simulink model "Model2"  (R2024b)
settings: Solver=ode4  StartTime=0.0  StopTime=100  FixedStep=0.01  RelTol=1e-3
values from neighbouring files (symbols this model uses):
  ARM_P_PID = [10 0 20]*0.1    [Single_ARM_Monte.m]    (also in main_starter.m)
  ARM_T_PID = [100 0 0]    [Single_ARM_Monte.m]    (also in main_starter.m)
  ARM_V_PID = [10 0 5]*0.1    [Single_ARM_Monte.m]    (also in main_starter.m)
  D_Joint0_angle0 = 45    [Single_ARM_Monte.m]    (also in main_starter.m)
  D_Joint0_angle1 = 0    [Single_ARM_Monte.m]    (also in main_starter.m)
  D_Joint0_angle2 = 0    [Single_ARM_Monte.m]    (also in main_starter.m)
  D_Joint0_rate0 = 0    [Single_ARM_Monte.m]    (also in main_starter.m)
  D_Joint0_rate1 = 0    [Single_ARM_Monte.m]    (also in main_starter.m)
  D_Joint0_rate2 = 0    [Single_ARM_Monte.m]    (also in main_starter.m)
  Joint_Motor_Mass = 23    [Single_ARM_Monte.m]    (also in main_starter.m)
  L_Joint0_angle0 = 45    [Single_ARM_Monte.m]    (also in main_starter.m)
  L_Joint0_angle1 = 0    [Single_ARM_Monte.m]    (also in main_starter.m)
  L_Joint0_angle2 = 0    [Single_ARM_Monte.m]    (also in main_starter.m)
  L_Joint0_rate0 = 0    [Single_ARM_Monte.m]    (also in main_starter.m)
  L_Joint0_rate1 = 0    [Single_ARM_Monte.m]    (also in main_starter.m)
  L_Joint0_rate2 = 0    [Single_ARM_Monte.m]    (also in main_starter.m)
  L_Joint_Offset = [ ... (first row only)    [Single_ARM_Monte.m]    (also in main_starter.m)
  Link1_Mass = 11    [Single_ARM_Monte.m]    (also in main_starter.m)
  Link2_Mass = 15.6    [Single_ARM_Monte.m]    (also in main_starter.m)
  Link3_Mass = 11    [Single_ARM_Monte.m]    (also in main_starter.m)
  Motor_transfer_Den = [1 100]    [Single_ARM_Monte.m]    (also in main_starter.m)
  Motor_transfer_Num = [100]    [Single_ARM_Monte.m]    (also in main_starter.m)
  PID_dt = 0.01    [Single_ARM_Monte.m]    (also in main_starter.m)
  R_Joint0_angle0 = 45    [Single_ARM_Monte.m]    (also in main_starter.m)
  R_Joint0_angle1 = 0    [Single_ARM_Monte.m]    (also in main_starter.m)
  R_Joint0_angle2 = 0    [Single_ARM_Monte.m]    (also in main_starter.m)
  R_Joint0_rate0 = 0    [Single_ARM_Monte.m]    (also in main_starter.m)
  R_Joint0_rate1 = 0    [Single_ARM_Monte.m]    (also in main_starter.m)
  R_Joint0_rate2 = 0    [Single_ARM_Monte.m]    (also in main_starter.m)
  RW_Att_D = 0.5    [Single_ARM_Monte.m]    (also in main_starter.m)
  RW_Att_I = 0.2    [Single_ARM_Monte.m]    (also in main_starter.m)
  RW_Att_P = 0.1    [Single_ARM_Monte.m]    (also in main_starter.m)
  RW_Mass = 100    [Single_ARM_Monte.m]    (also in main_starter.m)
  S_Body_Mass = 5    [Single_ARM_Monte.m]    (also in main_starter.m)
  S_init_pos = [0 0 0]'    [Single_ARM_Monte.m]    (also in main_starter.m)
  S_init_vel = [0 0 0]'    [Single_ARM_Monte.m]    (also in main_starter.m)
  T_Body_Mass = 4    [Single_ARM_Monte.m]    (also in main_starter.m)
  T_init_pos = [T_init_pos_list(i,1) T_init_pos_list(i,2) 0]'    [Single_ARM_Monte.m]    (also in main_starter.m = [1 0 0]')
  T_init_vel = [0 0 0]'    [Single_ARM_Monte.m]    (also in main_starter.m)
  Torq_mea_transfer_Den = [1 5]    [Single_ARM_Monte.m]    (also in main_starter.m)
  Torq_mea_transfer_Num = [5]    [Single_ARM_Monte.m]    (also in main_starter.m)
  U_Joint0_angle0 = 45    [Single_ARM_Monte.m]    (also in main_starter.m)
  U_Joint0_angle1 = 0    [Single_ARM_Monte.m]    (also in main_starter.m)
  U_Joint0_angle2 = 0    [Single_ARM_Monte.m]    (also in main_starter.m)
  U_Joint0_rate0 = 0    [Single_ARM_Monte.m]    (also in main_starter.m)
  U_Joint0_rate1 = 0    [Single_ARM_Monte.m]    (also in main_starter.m)
  U_Joint0_rate2 = 0    [Single_ARM_Monte.m]    (also in main_starter.m)
undefined symbols (not defined in the file or in its folder): X, Y, Z
libraries: nesl_utility x315, sm_lib x282, simulink_extras x46, sharedtransform x25, aerolibutil x4, simulink x2, matrix_library x2, dspmtrx3 x1
(part 12 of 12)

== matlab function Model2/Quad_ARM_Simplify/Down_ARM/MATLAB Function6 ==
  settings: updateMethod=DISCRETE
  data: cmd input; t_cmd output; cmd_d input; t_mea input; vd_mea input; v_mea input; p_mea input; mode input; tc_gain input; vc_gain input; pc_gain input; dt input
function t_cmd = motor_control(cmd,cmd_d, t_mea, vd_mea, v_mea, p_mea, mode, tc_gain, vc_gain, pc_gain, dt)

persistent I_save
persistent first_flg

if isempty(first_flg)
    I_save = 0;
    first_flg = 1;
end

if(mode == 1)%torque control
    % cmd : torque command [Nm]
    kp = tc_gain(1);
    ki = tc_gain(2);
    err = cmd - t_mea;
    t_cmd = kp*(cmd - t_mea) + ki*I_save;
    I_save = I_save + err*dt;

elseif(mode == 2) %velocity control
    % cmd : velocity command [rad/s]
    kp = vc_gain(1);
    % ki = vc_gain(2);
    kd = vc_gain(3);

    err = cmd - v_mea;
    errd = cmd_d - vd_mea;
    % t_cmd = (kp*err) + (kd*errd);
    t_cmd = (kp*err) + (kd*errd);
elseif(mode == 3) %position control : position command [rad]
    kp = pc_gain(1);
    % ki = pc_gain(2);
    kd = pc_gain(3);

    err = cmd - p_mea;
    errd = cmd_d - v_mea;
    t_cmd = (kp*err) + (kd*errd);
else%torque control
    t_cmd = 0;
end



end

== matlab function Model2/Quad_ARM_Simplify/Down_ARM/MATLAB Function7 ==
  data: v_sig input; v_out output; vd_out output; vd_sig input; t_mea input
function [v_out, vd_out] = limit_checker(v_sig,vd_sig,  t_mea)


if(abs(t_mea)>=0.01)
    vd_out = 0;
    v_out = 0;
else
    vd_out = vd_sig;
    v_out = v_sig;
end




end

== matlab function Model2/Quad_ARM_Simplify/End_Position_Flg ==
  data: L_J input; res output; R_J input; U_J input; D_J input
function res  = Motion_CMD(L_J, R_J, U_J, D_J)

deg2rad = 0.017453292519943;
rad2deg = 57.295779513082323;

L_END_FLG = 0;
R_END_FLG = 0;
U_END_FLG = 0;
D_END_FLG = 0;

Limit_Angle0 =     9.425*deg2rad;
Limit_Angle1 =   71.133*deg2rad;
Limit_Angle2 = 106.792*deg2rad;


L_END_FLG = End_Checker(L_J, [Limit_Angle0,-Limit_Angle1,-Limit_Angle2]);
R_END_FLG = End_Checker(R_J, [-Limit_Angle0,Limit_Angle1,Limit_Angle2]);
U_END_FLG = End_Checker(U_J, [-Limit_Angle0,Limit_Angle1,Limit_Angle2]);
D_END_FLG = End_Checker(D_J, [Limit_Angle0,-Limit_Angle1,-Limit_Angle2]);

res = [L_END_FLG,R_END_FLG,U_END_FLG,D_END_FLG]';

end

function res = End_Checker (Joint_Angle, Limit_Angle)

Limit_J0 = Limit_Angle(1);
Limit_J1 = Limit_Angle(2);
Limit_J2 = Limit_Angle(3);

J0 = Joint_Angle(1);
J1 = Joint_Angle(2);
J2 = Joint_Angle(3);

del = 5*pi/180;

J0_flg = 0; J1_flg = 0; J2_flg = 0;

if ((J0 <= (Limit_J0+del)) && (J0 >= (Limit_J0-del)))
    J0_flg = 1;
else
    J0_flg = 0;
end

if ((J1 <= (Limit_J1+del)) && (J1 >= (Limit_J1-del)))
    J1_flg = 1;
else
    J1_flg = 0;
end

if ((J2 <= (Limit_J2+del)) && (J2 >= (Limit_J2-del)))
    J2_flg = 1;
else
    J2_flg = 0;
end

if (J0_flg && J1_flg && J2_flg)
    res = 1;
else
    res = 0;
end

end

== matlab function Model2/Quad_ARM_Simplify/Fabrik_based_EE_Control(Angle) ==
  data: target input; q_list output; tol input; pos_list output; max_iter input; iter_fin output
function [q_list, pos_list, iter_fin] = fabrik_3link(target, tol, max_iter)
% target: [x; y] 목표 위치
% L: [L1, L2, L3] 링크 길이
% tol: 허용 오차 (예: 1e-4)
% max_iter: 반복 한계 (예: 100)

L = ...
[sqrt(0.04494^2 + 0.08979^2);
 0.1665;
 sqrt(0.02945^2 + 0.1232^2)];


[positions, ee_pose] = fk_3link([50,0,0]'*pi/180, L(1), L(2), L(3));

% 초기 관절 위치 (x, y) 초기화
pos_list = zeros(2, 4); % P0, P1, P2, P3
pos_list(:,1) = [0; 0];                    % Base
pos_list(:,2) = positions(:,1) + [L(1); 0]; % P1
pos_list(:,3) = positions(:,2) + [L(2); 0]; % P2
pos_list(:,4) = positions(:,3) + [L(3); 0]; % EE (초기화)

% Base 저장
base = pos_list(:,1);

% 목표 거리
total_length = sum(L);
if norm(target - base) > total_length
    % error("목표가 작업공간을 벗어났습니다.");
    target = total_length*(target/norm(target));
end

iter_fin = 0;

for iter = 1:max_iter
    % 1. FORWARD REACHING
    pos_list(:,4) = target; % 끝단 고정
    for i = 3:-1:1
        r = norm(pos_list(:,i+1) - pos_list(:,i));
        lambda = L(i) / r;
        pos_list(:,i) = (1 - lambda) * pos_list(:,i+1) + lambda * pos_list(:,i);
    end

    % 2. BACKWARD REACHING
    pos_list(:,1) = base; % base 고정
    for i = 1:3
        r = norm(pos_list(:,i+1) - pos_list(:,i));
        lambda = L(i) / r;
        pos_list(:,i+1) = (1 - lambda) * pos_list(:,i) + lambda * pos_list(:,i+1);
    end

    % 3. 수렴 확인
    err = norm(pos_list(:,end) - target);
    if err < tol
        break;
    end
    iter_fin = iter;
end

% P0 = joint_pos(:,1); P1 = joint_pos(:,2);
P2 = pos_list(:,2); P3 = pos_list(:,3);
% P4 = joint_pos(:,5); 
P5 = pos_list(:,4);

t0 = atan2(P2(2), P2(1));
temp = P3 - P2;
t1 = atan2(temp(2), temp(1)) - t0;
temp = P5 - P3;
t2 = atan2(temp(2), temp(1)) - t0 - t1;



q_list = [t0,t1,t2]';

end

function [positions, ee_pose] = fk_3link(theta, a1, a2, a3)
    % theta: [theta1, theta2, theta3] (rad)
    % a1, a2, a3: 링크 길이
    % positions: [P0; P1; P2; P3] (각 조인트 위치)
    % ee_pose: [x, y, phi] (EE 위치 + 자세)

    theta1 = theta(1);
    theta2 = theta(2);
    theta3 = theta(3);

    % 누적 각도
    t1 = theta1;
    t2 = theta1 + theta2;
    t3 = t2 + theta3;

    % 각 조인트 위치 계산
    P0 = [0; 0];
    P1 = P0 + a1 * [cos(t1); sin(t1)];
    P2 = P1 + a2 * [cos(t2); sin(t2)];
    P3 = P2 + a3 * [cos(t3); sin(t3)];

    % 자세
    phi = t3;

    % 출력
    positions = [P0, P1, P2, P3];  % 각 열이 각 위치
    ee_pose = [P3(1), P3(2)]'; % EE 위치 및 방향
end

== matlab function Model2/Single_ARM/MATLAB Function ==
  data: theta input; pos output
function pos = fk_3link_explicit(theta)
    L0 = 0.04494;
    L1 = 0.08979;
    L2 = 0.1665;
    L3a = 0.02945;
    L3b = 0.1232;

    t0 = theta(1);
    t1 = theta(2);
    t2 = theta(3);
    t01 = t0 + t1;
    t012 = t01 + t2;

    R = @(theta) [cos(theta); sin(theta)];

    P0 = [0; 0];
    P1 = P0 + L0 * R(t0 + pi/2);
    P2 = P1 + L1 * R(t0);
    P3 = P2 + L2 * R(t01);
    P4 = P3 + L3a * R(t012 + pi/2);
    pos = P4 + L3b * R(t012);  % EE 위치
end

== matlab function Model2/Quad_ARM_Simplify/Jacobian_based_EE_Control(Rate) ==
  data: q input; qd_cmd output; target_pos input
function qd_cmd = Jacobian_based_EE_Control(q, target_pos)
% target_pos = [0.3 0 0]';
pos = fk_3link_explicit(q);
J = jacobian_3link(q);

L = ...
[sqrt(0.04494^2 + 0.08979^2);
 0.1665;
 sqrt(0.02945^2 + 0.1232^2)];

% 목표 거리
total_length = sum(L);
if norm(target_pos) > total_length
    % error("목표가 작업공간을 벗어났습니다.");
    target_pos = total_length*(target_pos/norm(target_pos));
end

err = 2*(target_pos - pos);
Z = 0*[1 1 1]';
qd_cmd = pinv(J)*err + (eye(3,3) - pinv(J)*J)*Z;

end

function pos = fk_3link_explicit(theta)
    L0 = 0.04494;
    L1 = 0.08979;
    L2 = 0.1665;
    L3a = 0.02945;
    L3b = 0.1232;

    t0 = theta(1);
    t1 = theta(2);
    t2 = theta(3);
    t01 = t0 + t1;
    t012 = t01 + t2;

    R = @(theta) [cos(theta); sin(theta)];

    P0 = [0; 0];
    P1 = P0 + L0 * R(t0 + pi/2);
    P2 = P1 + L1 * R(t0);
    P3 = P2 + L2 * R(t01);
    P4 = P3 + L3a * R(t012 + pi/2);
    pos = P4 + L3b * R(t012);  % EE 위치
end

function J = jacobian_3link(theta)
    L0 = 0.04494;
    L1 = 0.08979;
    L2 = 0.1665;
    L3a = 0.02945;
    L3b = 0.1232;

    t0 = theta(1);
    t1 = theta(2);
    t2 = theta(3);
    t01 = t0 + t1;
    t012 = t01 + t2;

    Rp = @(theta) [-sin(theta); cos(theta)]; 

    J1 =  L0 * Rp(t0 + pi/2) ...
         +L1 * Rp(t0) ...
         +L2 * Rp(t01) ...
         +L3a * Rp(t012 + pi/2) ...
         +L3b * Rp(t012);

    J2 =  L2 * Rp(t01) ...
         +L3a * Rp(t012 + pi/2) ...
         +L3b * Rp(t012);

    J3 =  L3a * Rp(t012 + pi/2) ...
         +L3b * Rp(t012);

    J = [J1, J2, J3];
end

== matlab function Model2/Quad_ARM_Simplify/Left_ARM/MATLAB Function2 ==
  settings: updateMethod=DISCRETE
  data: cmd input; t_cmd output; cmd_d input; t_mea input; vd_mea input; v_mea input; p_mea input; mode input; tc_gain input; vc_gain input; pc_gain input; dt input
function t_cmd = motor_control(cmd, cmd_d, t_mea, vd_mea, v_mea, p_mea, mode, tc_gain, vc_gain, pc_gain, dt)

persistent I_save
persistent first_flg

if isempty(first_flg)
    I_save = 0;
    first_flg = 1;
end

if(mode == 1)%torque control
    % cmd : torque command [Nm]
    kp = tc_gain(1);
    ki = tc_gain(2);
    err = cmd - t_mea;
    t_cmd = kp*(cmd - t_mea) + ki*I_save;
    I_save = I_save + err*dt;

elseif(mode == 2) %velocity control
    % cmd : velocity command [rad/s]
    kp = vc_gain(1);
    % ki = vc_gain(2);
    kd = vc_gain(3);

    err = cmd - v_mea;
    errd = cmd_d - vd_mea;
    % t_cmd = (kp*err) + (kd*errd);
    t_cmd = (kp*err) + (kd*errd);
elseif(mode == 3) %position control : position command [rad]
    kp = pc_gain(1);
    % ki = pc_gain(2);
    kd = pc_gain(3);

    err = cmd - p_mea;
    errd = cmd_d - v_mea;
    t_cmd = (kp*err) + (kd*errd);
else%torque control
    t_cmd = 0;
end



end

== matlab function Model2/Quad_ARM_Simplify/Left_ARM/MATLAB Function3 ==
  data: v_sig input; v_out output; vd_out output; vd_sig input; t_mea input
function [v_out, vd_out] = limit_checker(v_sig,vd_sig,  t_mea)


if(abs(t_mea)>=0.01)
    vd_out = 0;
    v_out = 0;
else
    vd_out = vd_sig;
    v_out = v_sig;
end




end

== matlab function Model2/Quad_ARM_Simplify/Left_ARM/MATLAB Function4 ==
  settings: updateMethod=DISCRETE
  data: cmd input; t_cmd output; cmd_d input; t_mea input; vd_mea input; v_mea input; p_mea input; mode input; tc_gain input; vc_gain input; pc_gain input; dt input
function t_cmd = motor_control(cmd,cmd_d, t_mea, vd_mea, v_mea, p_mea, mode, tc_gain, vc_gain, pc_gain, dt)

persistent I_save
persistent first_flg

if isempty(first_flg)
    I_save = 0;
    first_flg = 1;
end

if(mode == 1)%torque control
    % cmd : torque command [Nm]
    kp = tc_gain(1);
    ki = tc_gain(2);
    err = cmd - t_mea;
    t_cmd = kp*(cmd - t_mea) + ki*I_save;
    I_save = I_save + err*dt;

elseif(mode == 2) %velocity control
    % cmd : velocity command [rad/s]
    kp = vc_gain(1);
    % ki = vc_gain(2);
    kd = vc_gain(3);

    err = cmd - v_mea;
    errd = cmd_d - vd_mea;
    % t_cmd = (kp*err) + (kd*errd);
    t_cmd = (kp*err) + (kd*errd);
elseif(mode == 3) %position control : position command [rad]
    kp = pc_gain(1);
    ki = pc_gain(2);
    kd = pc_gain(3);

    err = cmd - p_mea;
    errd = cmd_d - v_mea;
    t_cmd = (kp*err) + (kd*errd);
else%torque control
    t_cmd = 0;
end



end

== matlab function Model2/Quad_ARM_Simplify/Left_ARM/MATLAB Function5 ==
  data: v_sig input; v_out output; vd_out output; vd_sig input; t_mea input
function [v_out, vd_out] = limit_checker(v_sig,vd_sig,  t_mea)


if(abs(t_mea)>=0.01)
    vd_out = 0;
    v_out = 0;
else
    vd_out = vd_sig;
    v_out = v_sig;
end




end

== matlab function Model2/Quad_ARM_Simplify/Left_ARM/MATLAB Function6 ==
  settings: updateMethod=DISCRETE
  data: cmd input; t_cmd output; cmd_d input; t_mea input; vd_mea input; v_mea input; p_mea input; mode input; tc_gain input; vc_gain input; pc_gain input; dt input
function t_cmd = motor_control(cmd,cmd_d, t_mea, vd_mea, v_mea, p_mea, mode, tc_gain, vc_gain, pc_gain, dt)

persistent I_save
persistent first_flg

if isempty(first_flg)
    I_save = 0;
    first_flg = 1;
end

if(mode == 1)%torque control
    % cmd : torque command [Nm]
    kp = tc_gain(1);
    ki = tc_gain(2);
    err = cmd - t_mea;
    t_cmd = kp*(cmd - t_mea) + ki*I_save;
    I_save = I_save + err*dt;

elseif(mode == 2) %velocity control
    % cmd : velocity command [rad/s]
    kp = vc_gain(1);
    % ki = vc_gain(2);
    kd = vc_gain(3);

    err = cmd - v_mea;
    errd = cmd_d - vd_mea;
    % t_cmd = (kp*err) + (kd*errd);
    t_cmd = (kp*err) + (kd*errd);
elseif(mode == 3) %position control : position command [rad]
    kp = pc_gain(1);
    % ki = pc_gain(2);
    kd = pc_gain(3);

    err = cmd - p_mea;
    errd = cmd_d - v_mea;
    t_cmd = (kp*err) + (kd*errd);
else%torque control
    t_cmd = 0;
end



end

== matlab function Model2/Single_ARM/MATLAB Function2 ==
  settings: updateMethod=DISCRETE
  data: cmd input; t_cmd output; cmd_d input; t_mea input; vd_mea input; v_mea input; p_mea input; mode input; tc_gain input; vc_gain input; pc_gain input; dt input
function t_cmd = motor_control(cmd,cmd_d, t_mea, vd_mea, v_mea, p_mea, mode, tc_gain, vc_gain, pc_gain, dt)

persistent I_save
persistent first_flg

if isempty(first_flg)
    I_save = 0;
    first_flg = 1;
end

if(mode == 1)%torque control
    % cmd : torque command [Nm]
    kp = tc_gain(1);
    ki = tc_gain(2);
    err = cmd - t_mea;
    t_cmd = kp*(cmd - t_mea) + ki*I_save;
    I_save = I_save + err*dt;

elseif(mode == 2) %velocity control
    % cmd : velocity command [rad/s]
    kp = vc_gain(1);
    % ki = vc_gain(2);
    kd = vc_gain(3);

    err = cmd - v_mea;
    errd = cmd_d - vd_mea;
    % t_cmd = (kp*err) + (kd*errd);
    t_cmd = (kp*err) + (kd*errd);
elseif(mode == 3) %position control : position command [rad]
    kp = pc_gain(1);
    % ki = pc_gain(2);
    kd = pc_gain(3);

    err = cmd - p_mea;
    errd = cmd_d - v_mea;
    t_cmd = (kp*err) + (kd*errd);
else%torque control
    t_cmd = 0;
end



end

== matlab function Model2/Quad_ARM_Simplify/Left_ARM/MATLAB Function7 ==
  data: v_sig input; v_out output; vd_out output; vd_sig input; t_mea input
function [v_out, vd_out] = limit_checker(v_sig,vd_sig,  t_mea)


if(abs(t_mea)>=0.01)
    vd_out = 0;
    v_out = 0;
else
    vd_out = vd_sig;
    v_out = v_sig;
end




end

== matlab function Model2/Quad_ARM_Simplify/MATLAB Function ==
  data: theta input; pos output
function pos = fk_3link_explicit(theta)
    L0 = 0.04494;
    L1 = 0.08979;
    L2 = 0.1665;
    L3a = 0.02945;
    L3b = 0.1232;

    t0 = theta(1);
    t1 = theta(2);
    t2 = theta(3);
    t01 = t0 + t1;
    t012 = t01 + t2;

    R = @(theta) [cos(theta); sin(theta)];

    P0 = [0; 0];
    P1 = P0 + L0 * R(t0 + pi/2);
    P2 = P1 + L1 * R(t0);
    P3 = P2 + L2 * R(t01);
    P4 = P3 + L3a * R(t012 + pi/2);
    pos = P4 + L3b * R(t012);  % EE 위치
end

== matlab function Model2/Quad_ARM_Simplify/MATLAB Function1 ==
  data: theta input; J output
function J = jacobian_3link(theta)
    L0 = 0.04494;
    L1 = 0.08979;
    L2 = 0.1665;
    L3a = 0.02945;
    L3b = 0.1232;

    t0 = theta(1);
    t1 = theta(2);
    t2 = theta(3);
    t01 = t0 + t1;
    t012 = t01 + t2;

    Rp = @(theta) [-sin(theta); cos(theta)]; 

    J1 =  L0 * Rp(t0 + pi/2) ...
         +L1 * Rp(t0) ...
         +L2 * Rp(t01) ...
         +L3a * Rp(t012 + pi/2) ...
         +L3b * Rp(t012);

    J2 =  L2 * Rp(t01) ...
         +L3a * Rp(t012 + pi/2) ...
         +L3b * Rp(t012);

    J3 =  L3a * Rp(t012 + pi/2) ...
         +L3b * Rp(t012);

    J = [J1, J2, J3];
end

== matlab function Model2/Quad_ARM_Simplify/MATLAB Function2 ==
  data: u input; y output
function y = fcn(u)

y = u(:,4);

end

== matlab function Model2/Quad_ARM_Simplify/MATLAB Function3 ==
  data: theta input; pos output
function pos = fk_3link_explicit(theta)
    L0 = 0.04494;
    L1 = 0.08979;
    L2 = 0.1665;
    L3a = 0.02945;
    L3b = 0.1232;

    t0 = theta(1);
    t1 = theta(2);
    t2 = theta(3);
    t01 = t0 + t1;
    t012 = t01 + t2;

    R = @(theta) [cos(theta); sin(theta)];

    P0 = [0; 0];
    P1 = P0 + L0 * R(t0 + pi/2);
    P2 = P1 + L1 * R(t0);
    P3 = P2 + L2 * R(t01);
    P4 = P3 + L3a * R(t012 + pi/2);
    pos = P4 + L3b * R(t012);  % EE 위치
end

== matlab function Model2/Quad_ARM_Simplify/MATLAB Function5 ==
  data: theta input; pos output
function pos = fk_3link_explicit(theta)
    L0 = 0.04494;
    L1 = 0.08979;
    L2 = 0.1665;
    L3a = 0.02945;
    L3b = 0.1232;

    t0 = theta(1);
    t1 = theta(2);
    t2 = theta(3);
    t01 = t0 + t1;
    t012 = t01 + t2;

    R = @(theta) [cos(theta); sin(theta)];

    P0 = [0; 0];
    P1 = P0 + L0 * R(t0 + pi/2);
    P2 = P1 + L1 * R(t0);
    P3 = P2 + L2 * R(t01);
    P4 = P3 + L3a * R(t012 + pi/2);
    pos = P4 + L3b * R(t012);  % EE 위치
end

== matlab function Model2/Quad_ARM_Simplify/MATLAB Function6 ==
  data: theta input; positions output; ee_pose output
function [positions, ee_pose] = fk_3link_simplify(theta)
    % theta: [theta1, theta2, theta3] (rad)
    % a1, a2, a3: 링크 길이
    % positions: [P0; P1; P2; P3] (각 조인트 위치)
    % ee_pose: [x, y, phi] (EE 위치 + 자세)

    L = [sqrt(0.04494^2 + 0.08979^2);
           0.1665;
           sqrt(0.02945^2 + 0.1232^2)];

    theta1 = theta(1);
    theta2 = theta(2);
    theta3 = theta(3);

    % 누적 각도
    t1 = theta1;
    t2 = theta1 + theta2;
    t3 = t2 + theta3;

    % 각 조인트 위치 계산
    P0 = [0; 0];
    P1 = P0 + L(1) * [cos(t1); sin(t1)];
    P2 = P1 + L(2) * [cos(t2); sin(t2)];
    P3 = P2 + L(3) * [cos(t3); sin(t3)];

    % 자세
    phi = t3;

    % 출력
    positions = [P0, P1, P2, P3];  % 각 열이 각 위치
    ee_pose = [P3(1), P3(2)]'; % EE 위치 및 방향
end

== matlab function Model2/Quad_ARM_Simplify/Openning_Motion_Sequence ==
  data: b_flg input; res output; mode output
function [res, mode] = Motion_CMD(b_flg)

deg2rad = pi/180;

% if (t <= 10)
%     res = [45 -90 -180]'*deg2rad;
% 
% elseif ((t>=10) && (t<=20))
%     res = [45 0 -180]'*deg2rad;
% else
%     res = [45 0 0]'*deg2rad;
% end
% 
% mode = [3 3 3]';

Body_Contact_Total = (b_flg(1) == 1) && (b_flg(2) == 1) && (b_flg(3) == 1) && (b_flg(4) == 1);

if Body_Contact_Total
    res = [0 0 0]'*deg2rad;
    mode = [2 2 2]';
else
    res = [-4 -3 -4]'*deg2rad;
    mode = [2 2 2]';
end

end

== matlab function Model2/Quad_ARM_Simplify/Openning_Motion_Sequence1 ==
  data: t input; res output; mode output
function [res, mode] = Motion_CMD(t)

deg2rad = pi/180;

if (t <= 10)
    res = [45 -90 -180]'*deg2rad;

elseif ((t>=10) && (t<=20))
    res = [45 0 -180]'*deg2rad;
else
    res = [45 0 0]'*deg2rad;
end

mode = [3 3 3]';

end

== matlab function Model2/Quad_ARM_Simplify/Openning_Motion_Sequence2 ==
  data: b_flg input; res output; mode output
function [res, mode] = Motion_CMD(b_flg)

deg2rad = pi/180;

% if (t <= 10)
%     res = [45 -90 -180]'*deg2rad;
% 
% elseif ((t>=10) && (t<=20))
%     res = [45 0 -180]'*deg2rad;
% else
%     res = [45 0 0]'*deg2rad;
% end
% 
% mode = [3 3 3]';
% res = [-4 -3 -4]'*deg2rad;
% mode = [2 2 2]';
% res = [45 0 0]'*deg2rad;
% mode = [3 3 3]';
% 

Body_Contact_Total = (b_flg(1) == 1) && (b_flg(2) == 1) && (b_flg(3) == 1) && (b_flg(4) == 1);

if Body_Contact_Total
    res = [0 0 0]'*deg2rad;
    mode = [2 2 2]';
else
    res = [-4 -3 -4]'*deg2rad;
    mode = [2 2 2]';
end


end

== matlab function Model2/Quad_ARM_Simplify/Openning_Motion_Sequence3 ==
  data: b_flg input; res output; mode output
function [res, mode] = Motion_CMD(b_flg)

deg2rad = pi/180;

% res = [45 0 0]'*deg2rad;
% mode = [3 3 3]';


Body_Contact_Total = (b_flg(1) == 1) && (b_flg(2) == 1) && (b_flg(3) == 1) && (b_flg(4) == 1);

if Body_Contact_Total
    res = [0 0 0]'*deg2rad;
    mode = [2 2 2]';
else
    res = [-4 -3 -4]'*deg2rad;
    mode = [2 2 2]';
end

end

== matlab function Model2/Quad_ARM_Simplify/Openning_Motion_Sequence4 ==
  data: b_flg input; res output; mode output; pos_end_flg input
function [res, mode] = Motion_CMD(b_flg, pos_end_flg)

deg2rad = pi/180;

% res = [0 0 0]'*deg2rad;
% mode = [3 3 3]';


Body_Contact_Total = (b_flg(1) == 1) && (b_flg(2) == 1) && (b_flg(3) == 1) && (b_flg(4) == 1);
Pos_End_Total = pos_end_flg(1) && pos_end_flg(2) && pos_end_flg(3) && pos_end_flg(4);


if (Body_Contact_Total || Pos_End_Total)
    res = [0 0 0]'*deg2rad;
    mode = [2 2 2]';
else
    res = [-1 -2 -3]'*deg2rad;
    mode = [2 2 2]';
end

end

== matlab function Model2/Quad_ARM_Simplify/Right_ARM/MATLAB Function2 ==
  settings: updateMethod=DISCRETE
  data: cmd input; t_cmd output; cmd_d input; t_mea input; vd_mea input; v_mea input; p_mea input; mode input; tc_gain input; vc_gain input; pc_gain input; dt input
function t_cmd = motor_control(cmd, cmd_d, t_mea, vd_mea, v_mea, p_mea, mode, tc_gain, vc_gain, pc_gain, dt)

persistent I_save
persistent first_flg

if isempty(first_flg)
    I_save = 0;
    first_flg = 1;
end

if(mode == 1)%torque control
    % cmd : torque command [Nm]
    kp = tc_gain(1);
    ki = tc_gain(2);
    err = cmd - t_mea;
    t_cmd = kp*(cmd - t_mea) + ki*I_save;
    I_save = I_save + err*dt;

elseif(mode == 2) %velocity control
    % cmd : velocity command [rad/s]
    kp = vc_gain(1);
    % ki = vc_gain(2);
    kd = vc_gain(3);

    err = cmd - v_mea;
    errd = cmd_d - vd_mea;
    % t_cmd = (kp*err) + (kd*errd);
    t_cmd = (kp*err) + (kd*errd);
elseif(mode == 3) %position control : position command [rad]
    kp = pc_gain(1);
    % ki = pc_gain(2);
    kd = pc_gain(3);

    err = cmd - p_mea;
    errd = cmd_d - v_mea;
    t_cmd = (kp*err) + (kd*errd);
else%torque control
    t_cmd = 0;
end



end

== matlab function Model2/Quad_ARM_Simplify/Right_ARM/MATLAB Function3 ==
  data: v_sig input; v_out output; vd_out output; vd_sig input; t_mea input
function [v_out, vd_out] = limit_checker(v_sig,vd_sig,  t_mea)


if(abs(t_mea)>=0.01)
    vd_out = 0;
    v_out = 0;
else
    vd_out = vd_sig;
    v_out = v_sig;
end




end

== matlab function Model2/Quad_ARM_Simplify/Right_ARM/MATLAB Function4 ==
  settings: updateMethod=DISCRETE
  data: cmd input; t_cmd output; cmd_d input; t_mea input; vd_mea input; v_mea input; p_mea input; mode input; tc_gain input; vc_gain input; pc_gain input; dt input
function t_cmd = motor_control(cmd,cmd_d, t_mea, vd_mea, v_mea, p_mea, mode, tc_gain, vc_gain, pc_gain, dt)

persistent I_save
persistent first_flg

if isempty(first_flg)
    I_save = 0;
    first_flg = 1;
end

if(mode == 1)%torque control
    % cmd : torque command [Nm]
    kp = tc_gain(1);
    ki = tc_gain(2);
    err = cmd - t_mea;
    t_cmd = kp*(cmd - t_mea) + ki*I_save;
    I_save = I_save + err*dt;

elseif(mode == 2) %velocity control
    % cmd : velocity command [rad/s]
    kp = vc_gain(1);
    % ki = vc_gain(2);
    kd = vc_gain(3);

    err = cmd - v_mea;
    errd = cmd_d - vd_mea;
    % t_cmd = (kp*err) + (kd*errd);
    t_cmd = (kp*err) + (kd*errd);
elseif(mode == 3) %position control : position command [rad]
    kp = pc_gain(1);
    ki = pc_gain(2);
    kd = pc_gain(3);

    err = cmd - p_mea;
    errd = cmd_d - v_mea;
    t_cmd = (kp*err) + (kd*errd);
else%torque control
    t_cmd = 0;
end



end

== matlab function Model2/Quad_ARM_Simplify/Right_ARM/MATLAB Function5 ==
  data: v_sig input; v_out output; vd_out output; vd_sig input; t_mea input
function [v_out, vd_out] = limit_checker(v_sig,vd_sig,  t_mea)


if(abs(t_mea)>=0.01)
    vd_out = 0;
    v_out = 0;
else
    vd_out = vd_sig;
    v_out = v_sig;
end




end

== matlab function Model2/Quad_ARM_Simplify/Right_ARM/MATLAB Function6 ==
  settings: updateMethod=DISCRETE
  data: cmd input; t_cmd output; cmd_d input; t_mea input; vd_mea input; v_mea input; p_mea input; mode input; tc_gain input; vc_gain input; pc_gain input; dt input
function t_cmd = motor_control(cmd,cmd_d, t_mea, vd_mea, v_mea, p_mea, mode, tc_gain, vc_gain, pc_gain, dt)

persistent I_save
persistent first_flg

if isempty(first_flg)
    I_save = 0;
    first_flg = 1;
end

if(mode == 1)%torque control
    % cmd : torque command [Nm]
    kp = tc_gain(1);
    ki = tc_gain(2);
    err = cmd - t_mea;
    t_cmd = kp*(cmd - t_mea) + ki*I_save;
    I_save = I_save + err*dt;

elseif(mode == 2) %velocity control
    % cmd : velocity command [rad/s]
    kp = vc_gain(1);
    % ki = vc_gain(2);
    kd = vc_gain(3);

    err = cmd - v_mea;
    errd = cmd_d - vd_mea;
    % t_cmd = (kp*err) + (kd*errd);
    t_cmd = (kp*err) + (kd*errd);
elseif(mode == 3) %position control : position command [rad]
    kp = pc_gain(1);
    % ki = pc_gain(2);
    kd = pc_gain(3);

    err = cmd - p_mea;
    errd = cmd_d - v_mea;
    t_cmd = (kp*err) + (kd*errd);
else%torque control
    t_cmd = 0;
end



end

== matlab function Model2/Single_ARM/MATLAB Function3 ==
  data: v_sig input; v_out output; vd_out output; vd_sig input; t_mea input
function [v_out, vd_out] = limit_checker(v_sig,vd_sig,  t_mea)


if(abs(t_mea)>=0.5)
    vd_out = 0;
    v_out = 0;
else
    vd_out = vd_sig;
    v_out = v_sig;
end




end

== matlab function Model2/Quad_ARM_Simplify/Right_ARM/MATLAB Function7 ==
  data: v_sig input; v_out output; vd_out output; vd_sig input; t_mea input
function [v_out, vd_out] = limit_checker(v_sig,vd_sig,  t_mea)


if(abs(t_mea)>=0.01)
    vd_out = 0;
    v_out = 0;
else
    vd_out = vd_sig;
    v_out = v_sig;
end




end

== matlab function Model2/Quad_ARM_Simplify/Subsystem1/MATLAB Function1 ==
  data: qe input; Omegad output; we input; P_gain input; I_gain input; D_gain input; RW_config input
function Omegad = fcn(qe, we, P_gain, I_gain, D_gain, RW_config)

deg2rad = pi/180;

% beta = 63*deg2rad;

% RW1_axis = [cos(beta), 0, -sin(beta)]';
% RW3_axis = [-cos(beta), 0, -sin(beta)]';
% RW2_axis = [0, -cos(beta), sin(beta)]';
% RW4_axis = [0,  cos(beta), sin(beta)]';
% 
% RW_config = [RW1_axis, RW2_axis, RW3_axis, RW4_axis];

Kp = P_gain*diag([1 1 1]);
Kd = D_gain*diag([1 1 1]);

t = -(Kp*[qe(2); qe(3); qe(4)] + Kd*we);

Omegad = pinv(RW_config) * t;

end

function res = Rzyx(z,y,x)
   res = Rz(z)*Ry(y)*Rx(x);
end

function res = Rx(a)
% % % ang : rad
res = [1 0 0;
       0 cos(a) sin(a);
       0 -sin(a) cos(a)];
end

function res = Ry(a)
% % % ang : rad

res = [cos(a) 0 -sin(a);
                  0 1 0;
          sin(a) 0 cos(a)];

end

function res = Rz(a)
% % % ang : rad
res = [cos(a) sin(a) 0;
       -sin(a) cos(a) 0;
       0 0 1];

end

== matlab function Model2/Quad_ARM_Simplify/Up_ARM/MATLAB Function2 ==
  settings: updateMethod=DISCRETE
  data: cmd input; t_cmd output; cmd_d input; t_mea input; vd_mea input; v_mea input; p_mea input; mode input; tc_gain input; vc_gain input; pc_gain input; dt input
function t_cmd = motor_control(cmd, cmd_d, t_mea, vd_mea, v_mea, p_mea, mode, tc_gain, vc_gain, pc_gain, dt)

persistent I_save
persistent first_flg

if isempty(first_flg)
    I_save = 0;
    first_flg = 1;
end

if(mode == 1)%torque control
    % cmd : torque command [Nm]
    kp = tc_gain(1);
    ki = tc_gain(2);
    err = cmd - t_mea;
    t_cmd = kp*(cmd - t_mea) + ki*I_save;
    I_save = I_save + err*dt;

elseif(mode == 2) %velocity control
    % cmd : velocity command [rad/s]
    kp = vc_gain(1);
    % ki = vc_gain(2);
    kd = vc_gain(3);

    err = cmd - v_mea;
    errd = cmd_d - vd_mea;
    % t_cmd = (kp*err) + (kd*errd);
    t_cmd = (kp*err) + (kd*errd);
elseif(mode == 3) %position control : position command [rad]
    kp = pc_gain(1);
    % ki = pc_gain(2);
    kd = pc_gain(3);

    err = cmd - p_mea;
    errd = cmd_d - v_mea;
    t_cmd = (kp*err) + (kd*errd);
else%torque control
    t_cmd = 0;
end



end

== matlab function Model2/Quad_ARM_Simplify/Up_ARM/MATLAB Function3 ==
  data: v_sig input; v_out output; vd_out output; vd_sig input; t_mea input
function [v_out, vd_out] = limit_checker(v_sig,vd_sig,  t_mea)


if(abs(t_mea)>=0.01)
    vd_out = 0;
    v_out = 0;
else
    vd_out = vd_sig;
    v_out = v_sig;
end




end

== matlab function Model2/Quad_ARM_Simplify/Up_ARM/MATLAB Function4 ==
  settings: updateMethod=DISCRETE
  data: cmd input; t_cmd output; cmd_d input; t_mea input; vd_mea input; v_mea input; p_mea input; mode input; tc_gain input; vc_gain input; pc_gain input; dt input
function t_cmd = motor_control(cmd,cmd_d, t_mea, vd_mea, v_mea, p_mea, mode, tc_gain, vc_gain, pc_gain, dt)

persistent I_save
persistent first_flg

if isempty(first_flg)
    I_save = 0;
    first_flg = 1;
end

if(mode == 1)%torque control
    % cmd : torque command [Nm]
    kp = tc_gain(1);
    ki = tc_gain(2);
    err = cmd - t_mea;
    t_cmd = kp*(cmd - t_mea) + ki*I_save;
    I_save = I_save + err*dt;

elseif(mode == 2) %velocity control
    % cmd : velocity command [rad/s]
    kp = vc_gain(1);
    % ki = vc_gain(2);
    kd = vc_gain(3);

    err = cmd - v_mea;
    errd = cmd_d - vd_mea;
    % t_cmd = (kp*err) + (kd*errd);
    t_cmd = (kp*err) + (kd*errd);
elseif(mode == 3) %position control : position command [rad]
    kp = pc_gain(1);
    ki = pc_gain(2);
    kd = pc_gain(3);

    err = cmd - p_mea;
    errd = cmd_d - v_mea;
    t_cmd = (kp*err) + (kd*errd);
else%torque control
    t_cmd = 0;
end



end

== matlab function Model2/Quad_ARM_Simplify/Up_ARM/MATLAB Function5 ==
  data: v_sig input; v_out output; vd_out output; vd_sig input; t_mea input
function [v_out, vd_out] = limit_checker(v_sig,vd_sig,  t_mea)


if(abs(t_mea)>=0.01)
    vd_out = 0;
    v_out = 0;
else
    vd_out = vd_sig;
    v_out = v_sig;
end




end

== matlab function Model2/Quad_ARM_Simplify/Up_ARM/MATLAB Function6 ==
  settings: updateMethod=DISCRETE
  data: cmd input; t_cmd output; cmd_d input; t_mea input; vd_mea input; v_mea input; p_mea input; mode input; tc_gain input; vc_gain input; pc_gain input; dt input
function t_cmd = motor_control(cmd,cmd_d, t_mea, vd_mea, v_mea, p_mea, mode, tc_gain, vc_gain, pc_gain, dt)

persistent I_save
persistent first_flg

if isempty(first_flg)
    I_save = 0;
    first_flg = 1;
end

if(mode == 1)%torque control
    % cmd : torque command [Nm]
    kp = tc_gain(1);
    ki = tc_gain(2);
    err = cmd - t_mea;
    t_cmd = kp*(cmd - t_mea) + ki*I_save;
    I_save = I_save + err*dt;

elseif(mode == 2) %velocity control
    % cmd : velocity command [rad/s]
    kp = vc_gain(1);
    % ki = vc_gain(2);
    kd = vc_gain(3);

    err = cmd - v_mea;
    errd = cmd_d - vd_mea;
    % t_cmd = (kp*err) + (kd*errd);
    t_cmd = (kp*err) + (kd*errd);
elseif(mode == 3) %position control : position command [rad]
    kp = pc_gain(1);
    % ki = pc_gain(2);
    kd = pc_gain(3);

    err = cmd - p_mea;
    errd = cmd_d - v_mea;
    t_cmd = (kp*err) + (kd*errd);
else%torque control
    t_cmd = 0;
end



end

== matlab function Model2/Single_ARM/MATLAB Function4 ==
  settings: updateMethod=DISCRETE
  data: cmd input; t_cmd output; cmd_d input; t_mea input; vd_mea input; v_mea input; p_mea input; mode input; tc_gain input; vc_gain input; pc_gain input; dt input
function t_cmd = motor_control(cmd,cmd_d, t_mea, vd_mea, v_mea, p_mea, mode, tc_gain, vc_gain, pc_gain, dt)

persistent I_save
persistent first_flg

if isempty(first_flg)
    I_save = 0;
    first_flg = 1;
end

if(mode == 1)%torque control
    % cmd : torque command [Nm]
    kp = tc_gain(1);
    ki = tc_gain(2);
    err = cmd - t_mea;
    t_cmd = kp*(cmd - t_mea) + ki*I_save;
    I_save = I_save + err*dt;

elseif(mode == 2) %velocity control
    % cmd : velocity command [rad/s]
    kp = vc_gain(1);
    % ki = vc_gain(2);
    kd = vc_gain(3);

    err = cmd - v_mea;
    errd = cmd_d - vd_mea;
    % t_cmd = (kp*err) + (kd*errd);
    t_cmd = (kp*err) + (kd*errd);
elseif(mode == 3) %position control : position command [rad]
    kp = pc_gain(1);
    % ki = pc_gain(2);
    kd = pc_gain(3);

    err = cmd - p_mea;
    errd = cmd_d - v_mea;
    t_cmd = (kp*err) + (kd*errd);
else%torque control
    t_cmd = 0;
end



end

== matlab function Model2/Quad_ARM_Simplify/Up_ARM/MATLAB Function7 ==
  data: v_sig input; v_out output; vd_out output; vd_sig input; t_mea input
function [v_out, vd_out] = limit_checker(v_sig,vd_sig,  t_mea)


if(abs(t_mea)>=0.01)
    vd_out = 0;
    v_out = 0;
else
    vd_out = vd_sig;
    v_out = v_sig;
end




end

== matlab function Model2/Single(Right)_ARM_Simplify/MATLAB Function7 ==
  settings: updateMethod=DISCRETE
  data: dTime output; elapsedTime input; differ_input output; input input
function [dTime, differ_input] = ex(elapsedTime, input)

    persistent pre_input 
    if isempty(pre_input)
        pre_input=0;
    end

    persistent pre_time 
    if isempty(pre_time)
        pre_time=0;
    end

    persistent sw
    if isempty(sw)
        sw=0;
    end

    differ_input=0;

    if (input>=0.1)
        if sw==0
            sw=1;
            pre_input = input;
            pre_time = elapsedTime;
        end
    end

    dTime = elapsedTime - pre_time;
    
    if ((dTime >=1.0)&&(sw==1))
        differ_input = (input - pre_input)/dTime;
        sw=0;
    end

end

== matlab function Model2/Single(Right)_ARM_Simplify/Subsystem/MATLAB Function8 ==
  data: EE_vel_J input; output output; flg output
function [output, flg] = fcn(EE_vel_J)

    persistent pre_EE_vel_J
    if isempty(pre_EE_vel_J)
        pre_EE_vel_J = zeros(2,1); 
    end

    max_threshold = 0.05;

    output = EE_vel_J(1) - pre_EE_vel_J(1);
    pre_EE_vel_J(1) = EE_vel_J(1);  

    if abs(EE_vel_J(1)) <= max_threshold
        flg = 1;
    else 
        flg = 0;
    end
end

== matlab function Model2/Single(Right)_ARM_Simplify/Subsystem1/MATLAB Function1 ==
  data: qe input; Omegad output; we input; P_gain input; I_gain input; D_gain input; RW_config input
function Omegad = fcn(qe, we, P_gain, I_gain, D_gain, RW_config)

deg2rad = pi/180;

% beta = 63*deg2rad;

% RW1_axis = [cos(beta), 0, -sin(beta)]';
% RW3_axis = [-cos(beta), 0, -sin(beta)]';
% RW2_axis = [0, -cos(beta), sin(beta)]';
% RW4_axis = [0,  cos(beta), sin(beta)]';
% 
% RW_config = [RW1_axis, RW2_axis, RW3_axis, RW4_axis];

Kp = P_gain*diag([1 1 1]);
Kd = D_gain*diag([1 1 1]);

t = -(Kp*[qe(2); qe(3); qe(4)] + Kd*we);

Omegad = pinv(RW_config) * t;

end

function res = Rzyx(z,y,x)
   res = Rz(z)*Ry(y)*Rx(x);
end

function res = Rx(a)
% % % ang : rad
res = [1 0 0;
       0 cos(a) sin(a);
       0 -sin(a) cos(a)];
end

function res = Ry(a)
% % % ang : rad

res = [cos(a) 0 -sin(a);
                  0 1 0;
          sin(a) 0 cos(a)];

end

function res = Rz(a)
% % % ang : rad
res = [cos(a) sin(a) 0;
       -sin(a) cos(a) 0;
       0 0 1];

end

== matlab function Model2/Single(Right)_ARM_Simplify/MATLAB Function11 ==
  data: slip_warning_flg input; system_overload output; system_slip_ing output; system_slip_confirm output; slip_confirm_flg input; Overload_flg input; touch_flg input; empty_flg input; RPos_3 input; system_empty output
function [system_overload, system_slip_ing, system_slip_confirm,system_empty] = sysstate(slip_warning_flg, slip_confirm_flg, ...
                                                                  Overload_flg, touch_flg, empty_flg ,RPos_3)

%%%%empty판별
if empty_flg ==1
    system_empty =1;
else
    system_empty=0;
end

%%%%slip판별
if slip_warning_flg ==1
    system_slip_ing =1;
else
    system_slip_ing=0;
end


if slip_confirm_flg ==1
    system_slip_confirm =1;
else
    system_slip_confirm=0;
end


%%%%overload판별

if Overload_flg ==1
    system_overload =1;
else
    system_overload=0;
end


end

== matlab function Model2/Single(Right)_ARM_Simplify/Overload ==
  data: R_jtc input; overload_flg output; overload_start input
function overload_flg = over(R_jtc,overload_start)

  joint0_curr_limit = 36e-3;
  joint1_curr_limit = 3e-3;
  joint2_curr_limit = 3e-3;

  joint_limit = [joint0_curr_limit,joint1_curr_limit,joint2_curr_limit];
  joint0_curr = [R_jtc(1)];
  joint1_curr = [R_jtc(2)];
  joint2_curr = [R_jtc(3)];
  overload_flg =0;

if overload_start ==1

    if joint0_curr>=joint_limit(1) || joint1_curr>=joint_limit(2) || joint2_curr>=joint_limit(3) 
    
           overload_flg = 1;
     else
           overload_flg = 0;
    end 

end


end

== matlab function Model2/Single(Right)_ARM_Simplify/Slip_current ==
  settings: updateMethod=DISCRETE
  data: R_jtc input; slip_warning_flg output; touch_flg input; slip_confirm_flg output; I_avg_now output; dI output; dI_flg output; abs_I_flg output
function [slip_warning_flg, slip_confirm_flg,I_avg_now,dI,dI_flg,abs_I_flg] = detect_slip_emb(R_jtc, touch_flg)

    % --- 파라미터 설정 ---
    near_zero_threshold = 2e-2;     
    slip_drop_threshold = 1e-4;  
    slip_is_threshold = 1e-06;
    window_size = 5;               

    persistent buf_I count 
    persistent prev_avg_I
    persistent slip_warning_latched


    if isempty(slip_warning_latched)
        slip_warning_latched = 0;
    end
  
    if isempty(buf_I)
        buf_I = zeros(window_size, 3); 
        count = 0;
        prev_avg_I = zeros(1,3);
    end

    % 슬라이딩 윈도우 업데이트
    buf_I = [buf_I(2:end, :); R_jtc'];  % 최근 값 push
    count = min(count + 1, window_size);

    % 평균 전류 계산
    I_avg_now = mean(buf_I, 1);       % [3*1]
    dI = I_avg_now - prev_avg_I;      % 변화량

    % 현재 평균 전류의 절대값 (슬립 수렴 확인용)
    I_abs = abs(I_avg_now);

    % 플래그 초기화
    slip_warning_flg = 0;
    slip_confirm_flg = 0;
    dI_flg = 0;
    abs_I_flg = 0;

    % 슬립 경고 판단
    % 
    % if all(dI > -slip_drop_threshold)
    %     dI_flg =1;
    % end
    % 
    % if all(I_abs > slip_is_threshold)
    %     abs_I_flg =1;
    % end


    if touch_flg == 1 && any(I_abs > slip_is_threshold)
        if all(dI > -slip_drop_threshold)
            slip_warning_flg = 1;
            slip_warning_latched = 1;
        end
    end
    
    % 슬립 확정 판단

    if slip_warning_latched && all(I_avg_now < slip_is_threshold)
        slip_confirm_flg = 1;
        slip_warning_latched = 0;  % reset
    end

    % 평균 전류 갱신
    prev_avg_I = I_avg_now;
end

== matlab function Model2/Single(Right)_ARM_Simplify/EE_R ==
  data: R_J input; RPos_0 output; RPos_1 output; RPos_2 output; RPos_3 output
function[RPos_0, RPos_1, RPos_2, RPos_3] = fcn(R_J)
Right_pos = [15 -15  0]';


rad2deg = 180/pi;
deg2rad = pi/180;

% R_j= deg2rad*[-45 0 0 ]';

a =     [ 20 15 10]; %[cm]
d =     [ 0 0.0 0.0]; %[rad]
alpha = deg2rad*[ 0 0.0 0.0];%[rad]


R_A0 = Base(Right_pos);
RPos_0 = R_A0(1:3,4);

R_A1 = R_A0*Rotz(R_J(1))*transz(d(1))*transx(a(1));
RPos_1 = R_A1(1:3,4);

R_A2 = R_A1*Rotz(R_J(2))*transz(d(2))*transx(a(2));
RPos_2 = R_A2(1:3,4);

R_A3 = R_A2*Rotz(R_J(3))*transz(d(2))*transx(a(3));
RPos_3 =R_A3(1:3,4); %%  EE 위치

end


function [base] = Base(pos)
base = [1, 0, 0, pos(1);
        0, 1, 0, pos(2);
        0, 0, 1, pos(3);
        0, 0, 0,     1];
end



function [Rz] = Rotz(theta)


Rz = [cos(theta), -sin(theta), 0,0;
      sin(theta),  cos(theta), 0,0;
               0,           0, 1,0;
               0,           0, 0,1];

end

function [Rx] = Rotx(theta)

Rx = [1,  0, 0,0;
      0,  cos(theta),  sin(theta),0;
      0, -sin(theta),  cos(theta),0;
      0,           0,           0,1];

end

function [Tx] = transx(a)
Tx = [1, 0, 0, a;
      0, 1, 0, 0;
      0, 0, 1, 0;
      0, 0, 0, 1];

end

function [Tz] = transz(d)
Tz = [1, 0, 0, 0;
      0, 1, 0, 0;
      0, 0, 1, d;
      0, 0, 0, 1];

end
